simulink model "aero_coeffs_test"  (R2025b)
settings: Solver=VariableStepAuto  StartTime=0.0  StopTime=10.0  RelTol=1e-3
settings Model: Creator=deepa  LastModifiedBy=deepa

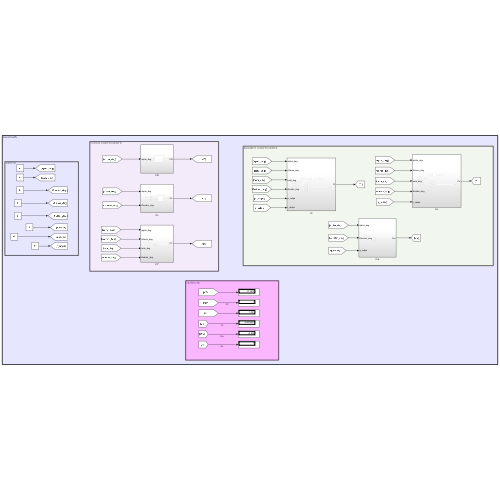
[thumbnail: Simulink's stored preview of the top-level diagram]
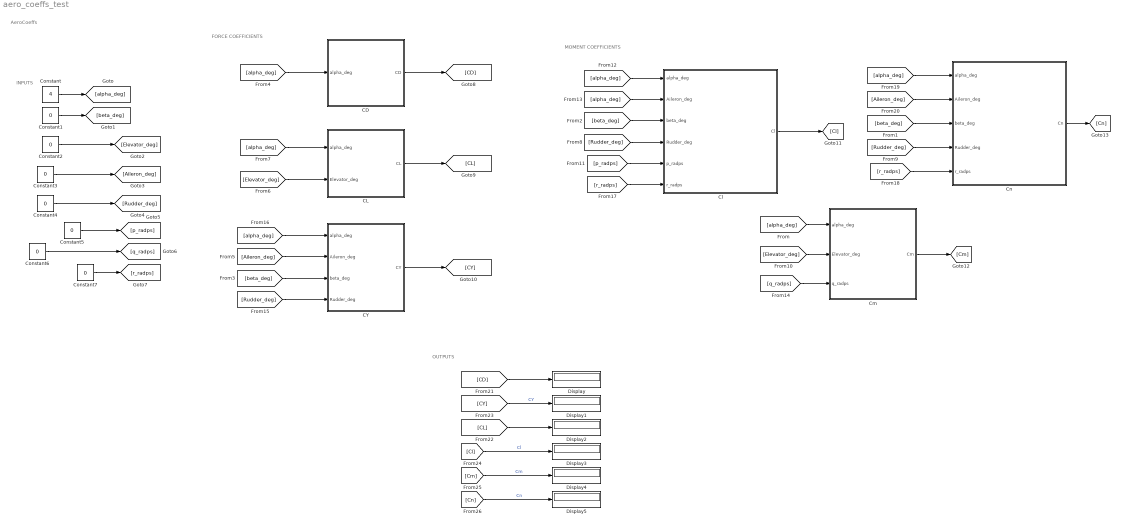
== system aero_coeffs_test ==
  note: AeroCoeffs
  note: OUTPUTS
  note: MOMENT COEFFICIENTS
  note: FORCE COEFFICIENTS
  note: INPUTS
  CD : Subsystem
  CL : Subsystem
  CY : Subsystem
  Cl : Subsystem
  Cm : Subsystem
  Cn : Subsystem
  Constant : Constant  Value=4
  Constant{1..7} (7 alike) : Constant  Value=0
  Display{,1..5} (6 alike) : Display
  wires:
  Constant4/1 -> [Rudder_deg]
  Constant3/1 -> [Aileron_deg]
  Constant2/1 -> [Elevator_deg]
  [alpha_deg] -> Cm/1(alpha_deg)
  [beta_deg] -> Cn/3(beta_deg)
  [beta_deg] -> Cl/3(beta_deg)
  [beta_deg] -> CY/3(beta_deg)
  [alpha_deg] -> CD/1(alpha_deg)
  [Aileron_deg] -> CY/2(Aileron_deg)
  [Elevator_deg] -> CL/2(Elevator_deg)
  [alpha_deg] -> CL/1(alpha_deg)
  [Rudder_deg] -> Cl/4(Rudder_deg)
  [Rudder_deg] -> Cn/4(Rudder_deg)
  [Elevator_deg] -> Cm/2(Elevator_deg)
  Constant5/1 -> [p_radps]
  Constant6/1 -> [q_radps]
  Constant7/1 -> [r_radps]
  [p_radps] -> Cl/5(p_radps)
  [alpha_deg] -> Cl/1(alpha_deg)
  [alpha_deg] -> Cl/2(Aileron_deg)
  [q_radps] -> Cm/3(q_radps)
  [Rudder_deg] -> CY/4(Rudder_deg)
  [alpha_deg] -> CY/1(alpha_deg)
  [r_radps] -> Cl/6(r_radps)
  [r_radps] -> Cn/5(r_radps)
  [alpha_deg] -> Cn/1(alpha_deg)
  [Aileron_deg] -> Cn/2(Aileron_deg)
  CD/1(CD) -> [CD]
  CL/1(CL) -> [CL]
  CY/1(CY) -> [CY]
  Cl/1(Cl) -> [Cl]
  Cm/1(Cm) -> [Cm]
  Cn/1(Cn) -> [Cn]
  [CD] -> Display/1
  [CY] -> Display1/1  "CY"
  [CL] -> Display2/1
  [Cn] -> Display5/1  "Cn"
  [Cm] -> Display4/1  "Cm"
  [Cl] -> Display3/1  "Cl"
  Constant/1 -> [alpha_deg]
  Constant1/1 -> [beta_deg]

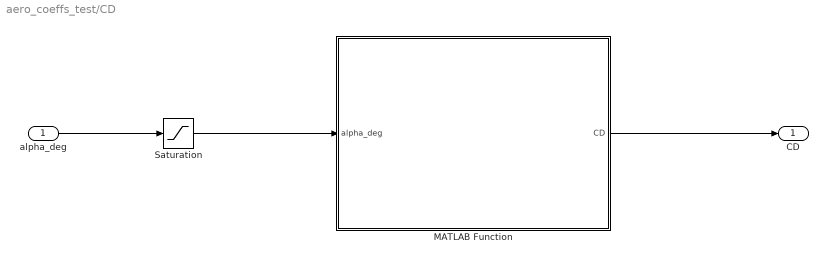
== system aero_coeffs_test/CD ==
  alpha_deg : Inport
  MATLAB Function : MATLAB Function  TreatAsAtomicUnit=on
  Saturation : Saturate  UpperLimit=40  LowerLimit=-5
  CD : Outport
  wires:
  Saturation/1 -> MATLAB Function/1(alpha_deg)
  MATLAB Function/1(CD) -> CD/1
  alpha_deg/1 -> Saturation/1

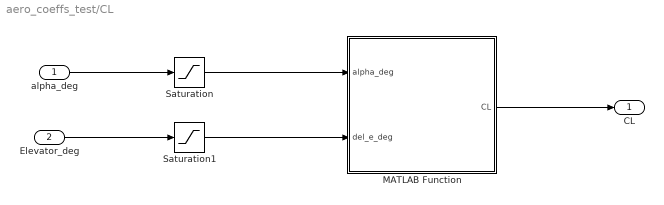
== system aero_coeffs_test/CL ==
  alpha_deg : Inport
  Elevator_deg : Inport  Port=2
  MATLAB Function : MATLAB Function  TreatAsAtomicUnit=on
  Saturation : Saturate  UpperLimit=40  LowerLimit=-5
  Saturation1 : Saturate  UpperLimit=30  LowerLimit=-30
  CL : Outport
  wires:
  MATLAB Function/1(CL) -> CL/1
  alpha_deg/1 -> Saturation/1
  Elevator_deg/1 -> Saturation1/1
  Saturation/1 -> MATLAB Function/1(alpha_deg)
  Saturation1/1 -> MATLAB Function/2(del_e_deg)

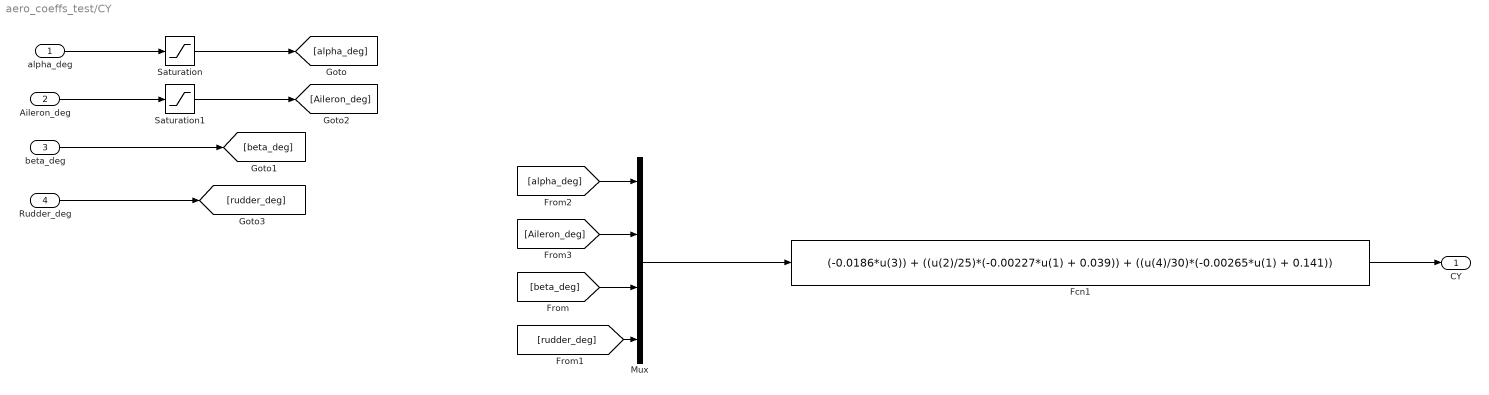
== system aero_coeffs_test/CY ==
  alpha_deg : Inport
  Aileron_deg : Inport  Port=2
  beta_deg : Inport  Port=3
  Rudder_deg : Inport  Port=4
  Fcn1 : Fcn  Expr=(-0.0186*u(3)) + ((u(2)/25)*(-0.00227*u(1) + 0.039)) + ((u(4)/30)*(-0.00265*u(1) + 0.141))
  Mux : Mux
  Saturation : Saturate  UpperLimit=35  LowerLimit=-5
  Saturation1 : Saturate  UpperLimit=40  LowerLimit=-5
  CY : Outport
  wires:
  [rudder_deg] -> Mux/4
  [beta_deg] -> Mux/3
  Rudder_deg/1 -> [rudder_deg]
  beta_deg/1 -> [beta_deg]
  Mux/1 -> Fcn1/1
  Saturation1/1 -> [Aileron_deg]
  Saturation/1 -> [alpha_deg]
  Fcn1/1 -> CY/1
  Aileron_deg/1 -> Saturation1/1
  alpha_deg/1 -> Saturation/1
  [alpha_deg] -> Mux/1
  [Aileron_deg] -> Mux/2

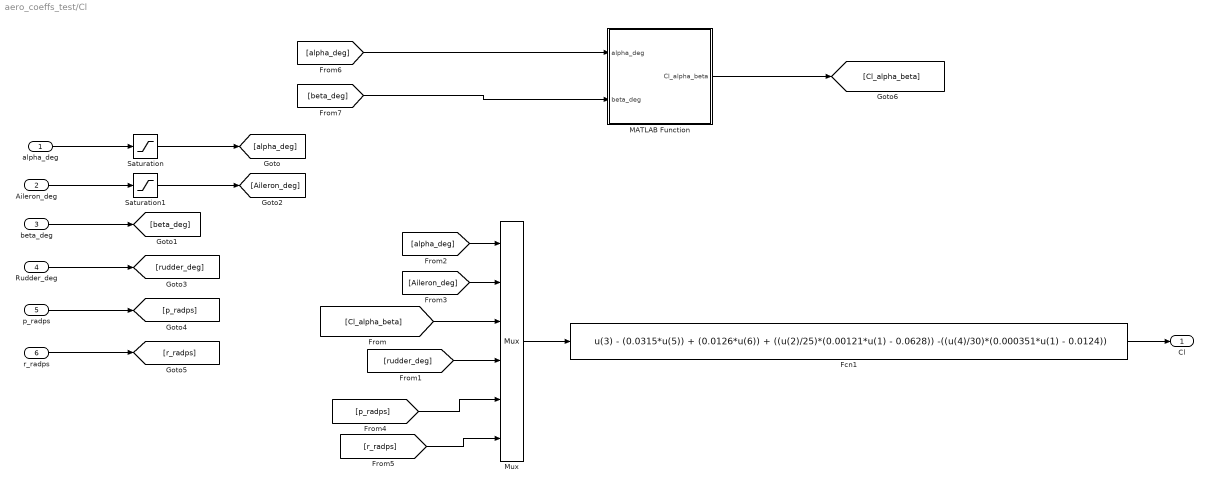
== system aero_coeffs_test/Cl ==
  alpha_deg : Inport
  Aileron_deg : Inport  Port=2
  beta_deg : Inport  Port=3
  Rudder_deg : Inport  Port=4
  p_radps : Inport  Port=5
  r_radps : Inport  Port=6
  Fcn1 : Fcn  Expr=u(3) - (0.0315*u(5)) + (0.0126*u(6)) + ((u(2)/25)*(0.00121*u(1) - 0.0628)) -((u(4)/30)*(0.000351*u(1) - 0.0124))
  MATLAB Function : MATLAB Function  TreatAsAtomicUnit=on
  Mux : Mux  Inputs=6
  Saturation : Saturate  UpperLimit=25  LowerLimit=-5
  Saturation1 : Saturate  UpperLimit=40  LowerLimit=-40
  Cl : Outport
  wires:
  MATLAB Function/1(Cl_alpha_beta) -> [Cl_alpha_beta]
  [alpha_deg] -> MATLAB Function/1(alpha_deg)
  [beta_deg] -> MATLAB Function/2(beta_deg)
  [r_radps] -> Mux/6
  [p_radps] -> Mux/5
  r_radps/1 -> [r_radps]
  p_radps/1 -> [p_radps]
  [Aileron_deg] -> Mux/2
  [alpha_deg] -> Mux/1
  alpha_deg/1 -> Saturation/1
  Aileron_deg/1 -> Saturation1/1
  Fcn1/1 -> Cl/1
  Saturation/1 -> [alpha_deg]
  Saturation1/1 -> [Aileron_deg]
  Mux/1 -> Fcn1/1
  beta_deg/1 -> [beta_deg]
  Rudder_deg/1 -> [rudder_deg]
  [Cl_alpha_beta] -> Mux/3
  [rudder_deg] -> Mux/4

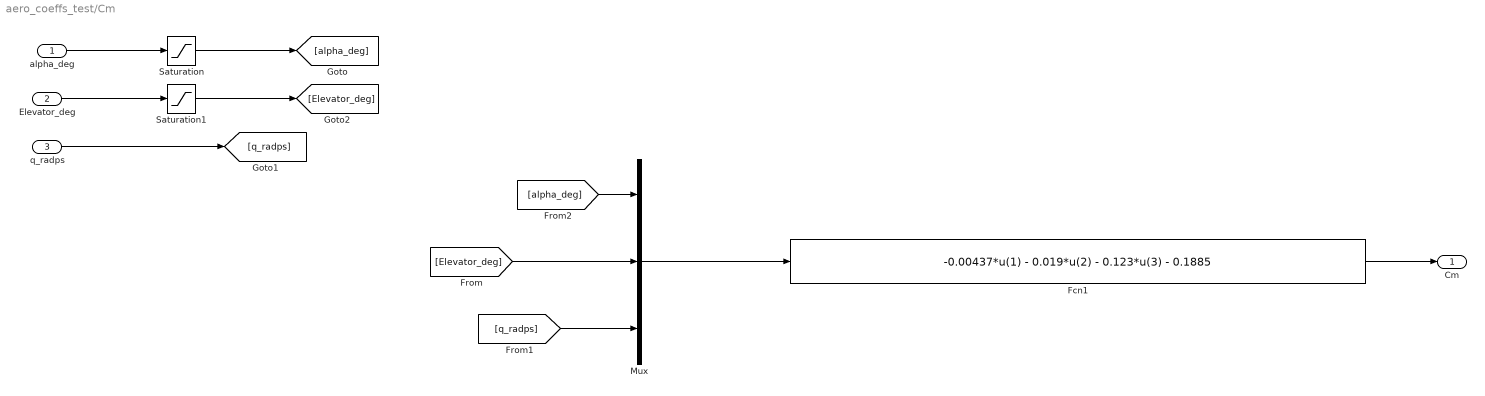
== system aero_coeffs_test/Cm ==
  alpha_deg : Inport
  Elevator_deg : Inport  Port=2
  q_radps : Inport  Port=3
  Fcn1 : Fcn  Expr=-0.00437*u(1) - 0.019*u(2) - 0.123*u(3) - 0.1885
  Mux : Mux  Inputs=3
  Saturation : Saturate  UpperLimit=40  LowerLimit=-5
  Saturation1 : Saturate  UpperLimit=40  LowerLimit=-5
  Cm : Outport
  wires:
  [q_radps] -> Mux/3
  [Elevator_deg] -> Mux/2
  [alpha_deg] -> Mux/1
  alpha_deg/1 -> Saturation/1
  Elevator_deg/1 -> Saturation1/1
  Fcn1/1 -> Cm/1
  Saturation/1 -> [alpha_deg]
  Saturation1/1 -> [Elevator_deg]
  Mux/1 -> Fcn1/1
  q_radps/1 -> [q_radps]

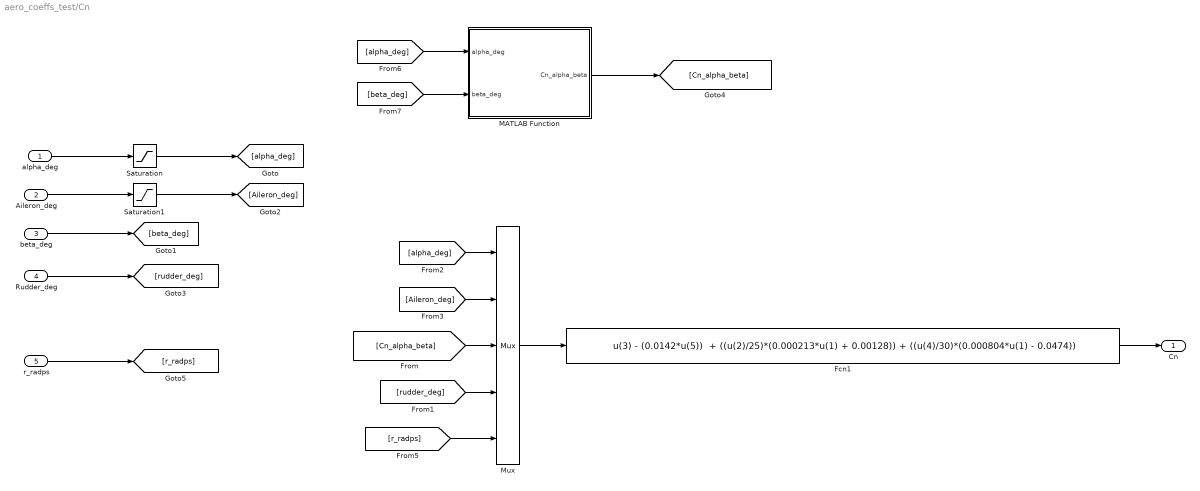
== system aero_coeffs_test/Cn ==
  alpha_deg : Inport
  Aileron_deg : Inport  Port=2
  beta_deg : Inport  Port=3
  Rudder_deg : Inport  Port=4
  r_radps : Inport  Port=5
  Fcn1 : Fcn  Expr="u(3) - (0.0142*u(5))  + ((u(2)/25)*(0.000213*u(1) + 0.00128)) + ((u(4)/30)*(0.000804*u(1) - 0.0474))"
  MATLAB Function : MATLAB Function  TreatAsAtomicUnit=on
  Mux : Mux  Inputs=5
  Saturation : Saturate  UpperLimit=35  LowerLimit=-5
  Saturation1 : Saturate  UpperLimit=40  LowerLimit=-5
  Cn : Outport
  wires:
  MATLAB Function/1(Cn_alpha_beta) -> [Cn_alpha_beta]
  [alpha_deg] -> MATLAB Function/1(alpha_deg)
  [rudder_deg] -> Mux/4
  [Cn_alpha_beta] -> Mux/3
  Rudder_deg/1 -> [rudder_deg]
  beta_deg/1 -> [beta_deg]
  Mux/1 -> Fcn1/1
  Saturation1/1 -> [Aileron_deg]
  Saturation/1 -> [alpha_deg]
  Fcn1/1 -> Cn/1
  Aileron_deg/1 -> Saturation1/1
  alpha_deg/1 -> Saturation/1
  [alpha_deg] -> Mux/1
  [Aileron_deg] -> Mux/2
  r_radps/1 -> [r_radps]
  [r_radps] -> Mux/5
  [beta_deg] -> MATLAB Function/2(beta_deg)

== matlab function aero_coeffs_test/CL/MATLAB Function ==
  data: alpha_deg input; CL output double; del_e_deg input
function  CL = fcn(alpha_deg, del_e_deg)

alpha = deg2rad(alpha_deg);
alpha0 = deg2rad(10);
delta = deg2rad(2);

w = 0.5*(1 + (tanh((alpha - alpha0)/delta)));

CL_low = 0.0752*alpha_deg + 0.0144*del_e_deg + 0.732;
CL_high = -0.00148*alpha_deg^2 - 0.106*alpha_deg + 0.0144*del_e_deg + 0.569;

CL = ((1-w)*CL_low) + (w*CL_high);

end

== matlab function aero_coeffs_test/Cl/MATLAB Function ==
  data: alpha_deg input; Cl_alpha_beta output; beta_deg input
function Cl_alpha_beta = fcn(alpha_deg, beta_deg)

alpha = deg2rad(alpha_deg);
alpha0 = deg2rad(15);
delta = deg2rad(2);

w = 0.5*(1 + (tanh((alpha - alpha0)/delta)));

Cl_alpha_beta_low = -0.00012*alpha_deg - 0.00092;
Cl_alpha_beta_high = 0.00022*alpha_deg - 0.006;

Cl_alpha_beta = beta_deg*((1-w)*Cl_alpha_beta_low + w*Cl_alpha_beta_high);

end

== matlab function aero_coeffs_test/Cn/MATLAB Function ==
  data: alpha_deg input; Cn_alpha_beta output; beta_deg input
function Cn_alpha_beta = fcn(alpha_deg, beta_deg)

Delta = deg2rad(2);   
alpha = deg2rad(alpha_deg);
w1 = 0.5*(1 + tanh((alpha - deg2rad(10))/Delta));
w2 = 0.5*(1 + tanh((alpha - deg2rad(25))/Delta));

% Regime models
f1 = 0.00125;
f2 = -0.00022*alpha + 0.00342;
f3 = -0.0020;

% Smooth combination
f_alpha = (1 - w1)*f1 + w1*(1 - w2)*f2 + w2*f3;

Cn_alpha_beta = beta_deg * f_alpha;
end

== matlab function aero_coeffs_test/CD/MATLAB Function ==
  data: alpha_deg input; CD output double
function CD = fcn(alpha_deg)

alpha = deg2rad(alpha_deg);
alpha0 = deg2rad(20);
delta = deg2rad(2);

w = 0.5*(1 + (tanh((alpha - alpha0)/delta)));

CD_low = -0.0000348*alpha_deg^2 + 0.0473*alpha_deg - 0.3358;
CD_high = 0.0013*alpha_deg^2 - 0.00438*alpha_deg + 0.1423;

CD = ((1-w)*CD_low) + (w*CD_high);

end
